simulink model "filter_quality_check_simple"  (R2014a)
settings: Solver=FixedStepDiscrete  StartTime=0.0  StopTime=inf  FixedStep=SampleTime  RelTol=1e-3
undefined symbols (not defined in the file or in its folder): SampleTime
settings Model: Creator=Jonas  LastModifiedBy=georg

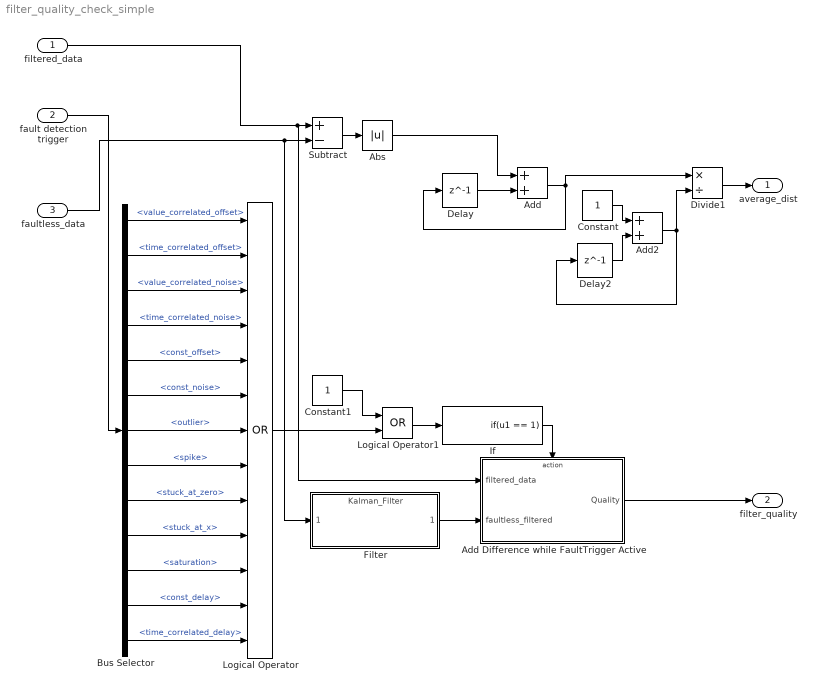
== system filter_quality_check_simple ==
  filtered_data : Inport
  fault detection trigger : Inport  Port=2  OutDataTypeStr=Bus: TriggerBus  SampleTime=SampleTime
  faultless_data : Inport  Port=3
  Abs : Abs
  Add : Sum
  Add Difference while FaultTrigger Active : Subsystem  TreatAsAtomicUnit=on
  Add2 : Sum
  Bus Selector : BusSelector  OutputSignals=value_correlated_offset,time_correlated_offset,value_correlated_noise,time_correlated_noise,const_offset,const_noise,outlier,spike,stuck_at_zero,stuck_at_x,saturation,const_delay,time_correlated_delay
  Constant : Constant
  Constant1 : Constant
  Delay : Delay  DelayLength=1  InitialCondition=0
  Delay2 : Delay  DelayLength=1  InitialCondition=0
  Divide1 : Product  Inputs=*/
  Filter : ModelReference  ModelNameDialog=Kalman_Filter.slx  SimulationMode=Normal  ModelReferenceVersion=1.2  CopyOfModelName=Kalman_Filter.slx  DefaultDataLogging=on
  If : If  IfExpression=u1 == 1  ShowElse=off
  Logical Operator : Logic  Operator=OR  Inputs=13  AllPortsSameDT=off  OutDataTypeStr=boolean
  Logical Operator1 : Logic  Operator=OR  AllPortsSameDT=off  OutDataTypeStr=boolean
  Subtract : Sum  Inputs=+-
  average_dist : Outport
  filter_quality : Outport  Port=2
  wires:
  filtered_data/1 -> Add Difference while FaultTrigger Active/1(filtered_data), Subtract/1
  faultless_data/1 -> Filter/1, Subtract/2
  Subtract/1 -> Abs/1
  Abs/1 -> Add/1
  Add/1 -> Divide1/1, Delay/1
  Delay/1 -> Add/2
  Divide1/1 -> average_dist/1
  Add2/1 -> Delay2/1, Divide1/2
  Delay2/1 -> Add2/2
  Constant/1 -> Add2/1
  fault detection trigger/1 -> Bus Selector/1
  Bus Selector/4 -> Logical Operator/4  "<time_correlated_noise>"
  Bus Selector/3 -> Logical Operator/3  "<value_correlated_noise>"
  Bus Selector/13 -> Logical Operator/13  "<time_correlated_delay>"
  Bus Selector/10 -> Logical Operator/10  "<stuck_at_x>"
  Bus Selector/11 -> Logical Operator/11  "<saturation>"
  Bus Selector/6 -> Logical Operator/6  "<const_noise>"
  Bus Selector/8 -> Logical Operator/8  "<spike>"
  Bus Selector/12 -> Logical Operator/12  "<const_delay>"
  Bus Selector/9 -> Logical Operator/9  "<stuck_at_zero>"
  Bus Selector/5 -> Logical Operator/5  "<const_offset>"
  Bus Selector/7 -> Logical Operator/7  "<outlier>"
  Bus Selector/2 -> Logical Operator/2  "<time_correlated_offset>"
  Bus Selector/1 -> Logical Operator/1  "<value_correlated_offset>"
  If/1 -> Add Difference while FaultTrigger Active/Action
  Add Difference while FaultTrigger Active/1(Quality) -> filter_quality/1
  Filter/1 -> Add Difference while FaultTrigger Active/2(faultless_filtered)
  Logical Operator/1 -> Logical Operator1/2
  Logical Operator1/1 -> If/1
  Constant1/1 -> Logical Operator1/1

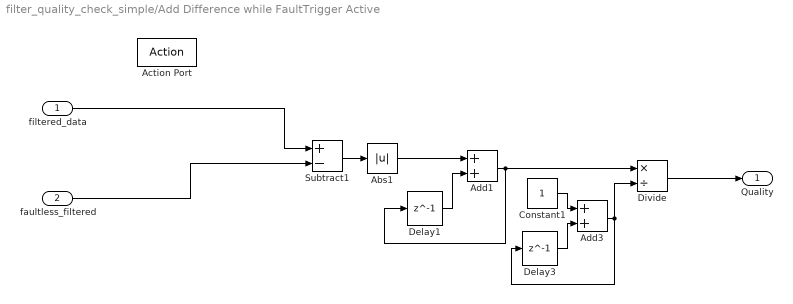
== system filter_quality_check_simple/Add Difference while FaultTrigger Active ==
  filtered_data : Inport
  faultless_filtered : Inport  Port=2
  Action Port : ActionPort  ActionType=then
  Abs1 : Abs
  Add1 : Sum
  Add3 : Sum
  Constant1 : Constant
  Delay1 : Delay  DelayLength=1  InitialCondition=0
  Delay3 : Delay  DelayLength=1  InitialCondition=0
  Divide : Product  Inputs=*/
  Subtract1 : Sum  Inputs=+-
  Quality : Outport
  wires:
  Subtract1/1 -> Abs1/1
  Abs1/1 -> Add1/1
  Add1/1 -> Divide/1, Delay1/1
  Delay1/1 -> Add1/2
  Divide/1 -> Quality/1
  Add3/1 -> Delay3/1, Divide/2
  Delay3/1 -> Add3/2
  Constant1/1 -> Add3/1
  faultless_filtered/1 -> Subtract1/2
  filtered_data/1 -> Subtract1/1
